simulink model "SynthFSE"  (R2023a)
settings: Solver=ode45  StartTime=0.0  StopTime=1780  RelTol=1e-3  EnableMultiTasking=on
undefined symbols (not defined in the file): j, QAM
libraries: hdlBasic x71, dspmlti4 x2, hdlUtilities x1, vmcUtilities x1
(part 1 of 2)
settings Model: Creator=alexc  LastModifiedBy=robg
settings SolverCC: AlgebraicLoopSolver=TrustRegion
settings DataIOCC: LimitDataPoints=on  SaveFormat=Array  SignalLoggingSaveFormat=ModelDataLogs  ReturnWorkspaceOutputs=off  SignalLoggingName=sigsOut
settings OptimizationCC: BlockReduction=off  BooleanDataType=off  ExpressionDepthLimit=2147483647  InitFltsAndDblsToZero=on  LifeSpan=inf
settings DebuggingCC: SaveWithParameterizedLinksMsg=none  UnderspecifiedInitializationDetection=Classic  MergeDetectMultiDrivingBlocksExec=none  SignalResolutionControl=TryResolveAllWithWarning  MultiTaskDSMMsg=warning  MultiTaskCondExecSysMsg=none  FcnCallInpInsideContextMsg=warning  UnconnectedInputMsg=warning  UnconnectedOutputMsg=warning  UnconnectedLineMsg=warning  StateNameClashWarn=warning  SFUnexpectedBacktrackingDiag=warning  SFNoUnconditionalDefaultTransitionDiag=warning  SFExecutionAtInitializationDiag=none  ArithmeticOperatorsInVariantConditions=warning
settings HardwareCC: ProdBitPerPointer=32  ProdBitPerSizeT=32  ProdBitPerPtrDiffT=32  ProdLargestAtomicFloat=None  ProdIntDivRoundTo=Undefined  ProdEndianess=Unspecified  ProdWordSize=32  ProdHWDeviceType=32-bit Generic  TargetUnknown=on
settings ModelReferenceCC: EnableRefExpFcnMdlSchedulingChecks=on  PropagateSignalLabelsOutOfModel=off
settings SFSimCC: SimUseLocalCustomCode=off  CustomCodeUndefinedFunction=UseInterfaceOnly
settings RTWCC: RTWUseLocalCustomCode=off  DLArmComputeVersion=19.05
settings CodeAppCC: StateflowObjectComments=on
settings GRTTargetCC: TargetFcnLib=ansi_tfl_tmw.mat  TargetLangStandard=C89/C90 (ANSI)  CombineOutputUpdateFcns=off  GRTInterface=on
settings ConfigComp: CovMetricSettings=dw  CovSaveCumulativeToWorkspaceVar=on  CovSaveSingleToWorkspaceVar=on  CovExternalEMLEnable=off

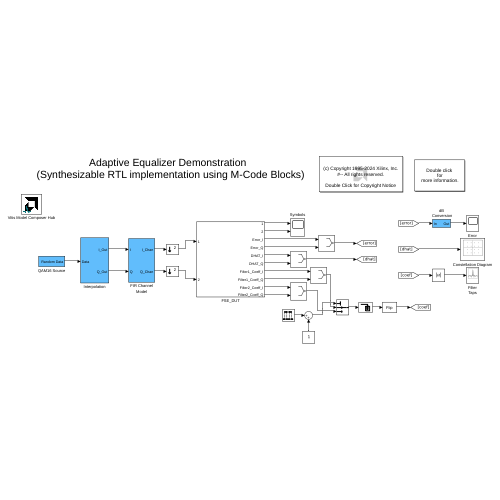
[thumbnail: Simulink's stored preview of the top-level diagram]
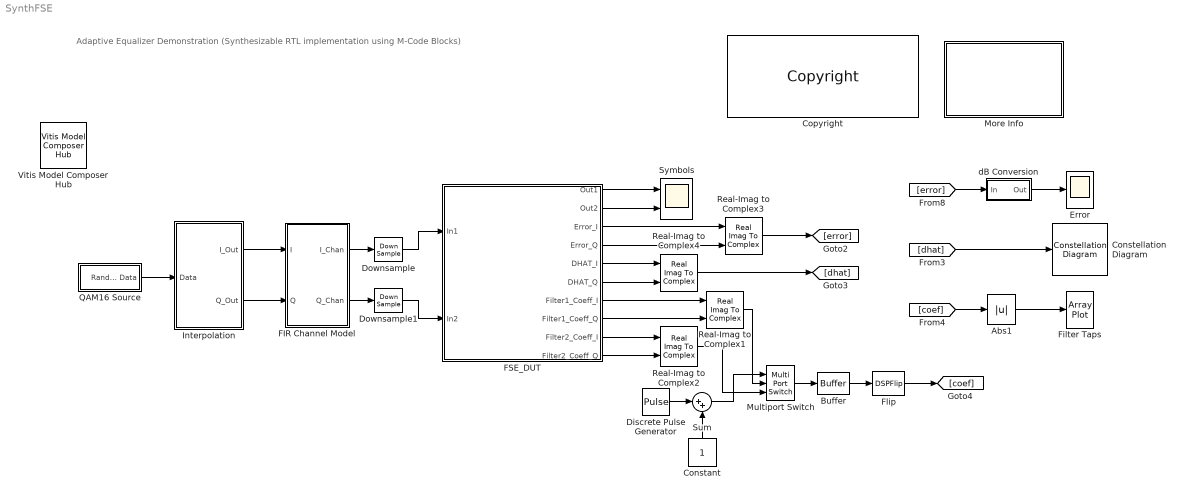
== system SynthFSE ==
  note: Adaptive Equalizer Demonstration
      | (Synthesizable RTL implementation using M-Code Blocks)
  Abs1 : Abs
  Buffer : Buffer  N=8
  Constant : Constant
  Constellation Diagram : ConstellationDiagram  WindowPosition=[288.000000,26.000000,474.000000,337.000000,]  ScopeFrameLocation=window  SymbolsToDisplaySource=Property  SymbolsToDisplay=1000  ReferenceConstellation=16-QAM  YLimits=[-1.8578 1.8744]  ColorFading=on  DefaultConfigurationName=comm.scopes.ConstellationDiagramBlockCfg
  Copyright : hdlUtilities/Copyright  copyrighttext="Copyright (c) 2024  by  Xilinx, Inc. All rights reserved.<br><br>This file contains proprietary, confidential information of Xilinx, Inc., is distributed under license from Xilinx, Inc., and may be used, copied and/or disclosed only pursuant to the terms of a valid license agreement with Xilinx, Inc. Xilinx hereby grants you a license to use this file solely for design, simulation, implementation and creation of design files limited to Xilinx devices or technologies. Use with non-Xilinx devices or technologies is expressly prohibited and immediately terminates your license unless covered by a separate agreement.<br><br>Xilinx is providing this design, code, or information \"as-is\" solely for use in developing programs and solutions for Xilinx devices, with no obligation on the part of Xilinx to provide support. By providing this design, code, or information as one possible implementation of this feature, application or standard, Xilinx is making no representation that this implementation is free from any claims of infringement. You are responsible for obtaining any rights you may require for your implementation. Xilinx expressly disclaims any warranty whatsoever with respect to the adequacy of the implementation, including but not limited to any warranties or representations that this implementation is free from claims of infringement, implied warranties of merchantability or fitness for a particular purpose.<br><br>Xilinx products are not intended for use in life support appliances, devices, or systems. Use in such applications is expressly prohibited.<br><br>Any modifications that are made to the Source Code are done at the user's sole risk and will be unsupported.<br><br>This copyright and support notice must be retained as part of this text at all times. (c) Copyright 1995-2024 Xilinx, Inc. All rights reserved."  block_type=copyright
  Discrete Pulse Generator : DiscretePulseGenerator  SampleTime=.5
  Downsample : DownSample  RateOptions=Allow multirate processing
  Downsample1 : DownSample  RateOptions=Allow multirate processing
  Error : Scope
  FIR Channel Model : Subsystem  mask{chan=[1+j*0.1 .2 j*0.2 0 0 0 0 0 0 0]}
      mask prompts: chan "Channel"
  FSE_DUT : Subsystem
  Filter Taps : ArrayPlot  WindowPosition=[66.000000,260.000000,329.000000,270.000000,]  ScopeFrameLocation=window  PlotType=Line  AxesScaling=Manual  MaximizeAxes=On  XLabel=Samples  YLabel=Filter Coefficients  YLimits=[0.005979,1.0369]  DefaultConfigurationName=dsp.scopes.ArrayPlotBlockSpecification
  Flip : DSPFlip
  Interpolation : Subsystem
  More Info : Subsystem
      mask Display: disp('Double click\n for\n more information.')
  Multiport Switch : MultiPortSwitch  Inputs=2
  QAM16 Source : Subsystem
  Real-Imag to Complex{1..4} (4 alike) : RealImagToComplex
  Sum : Sum  Inputs=|++  InputSameDT=on  SaturateOnIntegerOverflow=on  OutDataTypeStr=Inherit: Same as first input
  Symbols : Scope  NumInputPorts=2
  Vitis Model Composer Hub : vmcUtilities/Vitis Model Composer Hub  Tag=genX  CodeGeneration=off  SubsystemName=FSE_DUT  CompilationType=HDLCompilation  SubsystemType=HDLNode  ExportTypeV2=IP Catalog  StartColumn=1  NumberOfColumns=1  TargetDirectory=./netlist  exportDesign=on  analyzeDesign=off  validateDesignOnHw=off  ExportType=System Generator  IpVendor=xilinx.com  IpLibrary=hls  IpVersion=1.0  IpHWLanguage=Verilog  AieCompilerOptions={}  AieSimulatorOptions={}  CreateTestbench=off  TestbenchStackSize=10  RunRtlSim=off  RunCSim=off  RunAieSim=off  AieSimTimeout=50000  RunAieSimProfiling=off  LaunchVitisAnalyzer=off  PlotOutput=off  RunX86Sim=off  X86SimTimeout=10  GenHwImage=off  GenLibadfXo=on  GenHwValidationCode=off  PlatformType=Not Specified  HwSystemType=Baremetal  HwValidationTarget=hw  ProjDevice=xcku11p-ffva1156-1-e  ProjDevicePart=xcku11p-ffva1156-1-e  SamplePeriod=-1  ClockFrequency=200  DataPathParallelism=1  xilinxfamily=kintexuplus  part=xcku11p  speed=-1-e  package=ffva1156  directory=./netlist/ip/FSE_DUT/src  testbench=off  incr_netlist=off  synthesis_tool=Vivado  clock_wrapper=Clock Enables  dbl_ovrd=According to Block Masks  dcm_input_clock_period=10  sysclk_period=10  simulink_period=1  eval_field=0  IPInfoJsonString="{\"DUTSubsystemName\":\"FSE_DUT\",\"HDLSubsystem\":{\"SubsystemName\":\"FSE_DUT\",\"IPName\":\"Subsystem\",\"IPLibrary\":\"VMC\",\"IPVendor\":\"User Company\",\"IPVersion\":\"1.0\",\"TargetDirectory\":\"./netlist\",\"SubsystemDir\":\"./netlist/ip/FSE_DUT\",\"FreqHz\":\"100000000\"},\"SubsystemTag\":\"HDLNode\"}"  LogFileName=/group/xcoswmktg2/robg/git/vmc_examples/Vitis_Model_Composer/Examples/HDL/Digital_Filtering/LMS_based_adaptive_Equalization_Synth_RTL/netlist/model_composer.log  NThreads=4  IPConfigFile=/tmp/vmctmp-robg/363/ipconfig.json
  dB Conversion : Subsystem
  wires:
  QAM16 Source/1(" Random Data") -> Interpolation/1(Data)
  Interpolation/2(Q_Out) -> FIR Channel Model/2(Q)
  Interpolation/1(I_Out) -> FIR Channel Model/1(I)
  FIR Channel Model/1(I_Chan) -> Downsample/1
  FIR Channel Model/2(Q_Chan) -> Downsample1/1
  Abs1/1 -> Filter Taps/1
  dB Conversion/1(Out) -> Error/1
  [coef] -> Abs1/1
  [dhat] -> Constellation Diagram/1
  [error] -> dB Conversion/1(In)
  Discrete Pulse Generator/1 -> Sum/1
  Multiport Switch/1 -> Buffer/1
  Flip/1 -> [coef]
  Real-Imag to Complex2/1 -> Multiport Switch/3
  Constant/1 -> Sum/2
  Buffer/1 -> Flip/1
  Sum/1 -> Multiport Switch/1
  Real-Imag to Complex1/1 -> Multiport Switch/2
  Real-Imag to Complex4/1 -> [dhat]
  Real-Imag to Complex3/1 -> [error]
  Downsample/1 -> FSE_DUT/1(In1)
  Downsample1/1 -> FSE_DUT/2(In2)
  FSE_DUT/1(Out1) -> Symbols/1
  FSE_DUT/2(Out2) -> Symbols/2
  FSE_DUT/3(Error_I) -> Real-Imag to Complex3/1
  FSE_DUT/4(Error_Q) -> Real-Imag to Complex3/2
  FSE_DUT/5(DHAT_I) -> Real-Imag to Complex4/1
  FSE_DUT/6(DHAT_Q) -> Real-Imag to Complex4/2
  FSE_DUT/7(Filter1_Coeff_I) -> Real-Imag to Complex1/1
  FSE_DUT/8(Filter1_Coeff_Q) -> Real-Imag to Complex1/2
  FSE_DUT/9(Filter2_Coeff_I) -> Real-Imag to Complex2/1
  FSE_DUT/10(Filter2_Coeff_Q) -> Real-Imag to Complex2/2

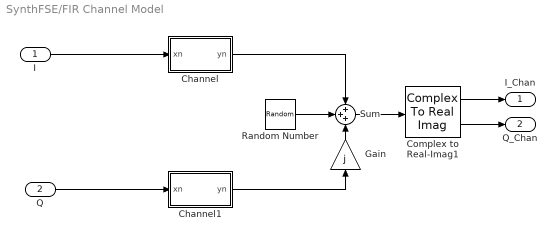
== system SynthFSE/FIR Channel Model ==
  I : Inport
  Q : Inport  Port=2
  Channel : Subsystem
  Channel1 : Subsystem
  Complex to Real-Imag1 : ComplexToRealImag
  Gain : Gain  Gain=j  SaturateOnIntegerOverflow=on  OutDataTypeStr=Inherit: Same as input  ParamDataTypeStr=Inherit: Same as input
  Random Number : RandomNumber  Variance=.01  SampleTime=100000
  Sum : Sum  Inputs=+++  InputSameDT=on  SaturateOnIntegerOverflow=on  OutDataTypeStr=Inherit: Same as first input
  I_Chan : Outport  VectorParamsAs1DForOutWhenUnconnected=off
  Q_Chan : Outport  Port=2  VectorParamsAs1DForOutWhenUnconnected=off
  wires:
  Channel1/1(yn) -> Gain/1
  Channel/1(yn) -> Sum/1
  Q/1 -> Channel1/1(xn)
  I/1 -> Channel/1(xn)
  Random Number/1 -> Sum/2
  Gain/1 -> Sum/3
  Sum/1 -> Complex to Real-Imag1/1
  Complex to Real-Imag1/2 -> Q_Chan/1
  Complex to Real-Imag1/1 -> I_Chan/1

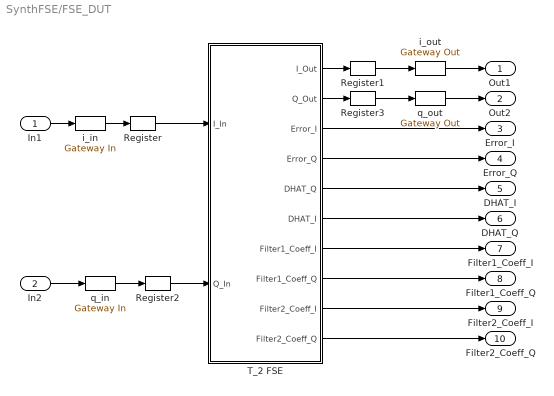
== system SynthFSE/FSE_DUT ==
  In1 : Inport
  In2 : Inport  Port=2
  Register{,1..3} (4 alike) : hdlBasic/Register  init=0  rst=off  en=off  XmcBlockStatus=1  maskContainerNames=tabcontainer1  block_type=register  block_config=sysgen:Register_config
  T_2 FSE : Subsystem  mask{mu=.005}
  i_in : hdlBasic/Gateway In  gui_display_data_type=Fixed-point  arith_type=Signed (2's comp)  n_bits=12  bin_pt=10  preci_type=Single  exp_width=8  frac_width=24  rows=1  columns=1  quantization="Round  (unbiased: +/- Inf)"  overflow=Saturate  period=2  UseAsADC=off  ADCChannel='1'  interface=None  automatic_assignment=on  address_offset=hex2dec('00')  intf_name=''  intf_description=''  default_value=0  timing_constraint=None  locs_specified=off  LOCs={}  io_standard={}  inherit_from_input=off  hdl_port=on  XmcBlockStatus=1  maskContainerNames=group4  block_type=gatewayin  block_config=sysgen:gateway_in_config  block_width_w=590  block_height_w=620  block_width=640  block_height=850
  i_out : hdlBasic/Gateway Out  inherit_from_input=off  hdl_port=on  rows=1  columns=1  UseAsDAC=off  DACChannel='1'  interface=None  automatic_assignment=on  address_offset=hex2dec('00')  intf_name=''  intf_description=''  timing_constraint="Data Rate;  Set 'FAST' Attribute"  locs_specified=off  LOCs={}  io_standard={}  XmcBlockStatus=1  maskContainerNames=group4  block_type=gatewayout  block_config=sysgen:gateway_out_config  block_width_w=590  block_height_w=620  block_width=620  block_height=750
  q_in : hdlBasic/Gateway In  gui_display_data_type=Fixed-point  arith_type=Signed (2's comp)  n_bits=12  bin_pt=10  preci_type=Single  exp_width=8  frac_width=24  rows=1  columns=1  quantization="Round  (unbiased: +/- Inf)"  overflow=Saturate  period=2  UseAsADC=off  ADCChannel='1'  interface=None  automatic_assignment=on  address_offset=hex2dec('00')  intf_name=''  intf_description=''  default_value=0  timing_constraint=None  locs_specified=off  LOCs={}  io_standard={}  inherit_from_input=off  hdl_port=on  XmcBlockStatus=1  maskContainerNames=group4  block_type=gatewayin  block_config=sysgen:gateway_in_config  block_width_w=590  block_height_w=620  block_width=640  block_height=850
  q_out : hdlBasic/Gateway Out  inherit_from_input=off  hdl_port=on  rows=1  columns=1  UseAsDAC=off  DACChannel='1'  interface=None  automatic_assignment=on  address_offset=hex2dec('00')  intf_name=''  intf_description=''  timing_constraint="Data Rate;  Set 'FAST' Attribute"  locs_specified=off  LOCs={}  io_standard={}  XmcBlockStatus=1  maskContainerNames=group4  block_type=gatewayout  block_config=sysgen:gateway_out_config  block_width_w=590  block_height_w=620  block_width=620  block_height=750
  Out1 : Outport
  Out2 : Outport  Port=2
  Error_I : Outport  Port=3
  Error_Q : Outport  Port=4
  DHAT_I : Outport  Port=5
  DHAT_Q : Outport  Port=6
  Filter1_Coeff_I : Outport  Port=7
  Filter1_Coeff_Q : Outport  Port=8
  Filter2_Coeff_I : Outport  Port=9
  Filter2_Coeff_Q : Outport  Port=10
  wires:
  T_2 FSE/5(DHAT_Q) -> DHAT_I/1
  Register/1 -> T_2 FSE/1(I_In)
  T_2 FSE/7(Filter1_Coeff_I) -> Filter1_Coeff_I/1
  T_2 FSE/8(Filter1_Coeff_Q) -> Filter1_Coeff_Q/1
  T_2 FSE/2(Q_Out) -> Register3/1
  Register3/1 -> q_out/1
  i_in/1 -> Register/1
  Register1/1 -> i_out/1
  T_2 FSE/3(Error_I) -> Error_I/1
  T_2 FSE/4(Error_Q) -> Error_Q/1
  q_out/1 -> Out2/1
  T_2 FSE/6(DHAT_I) -> DHAT_Q/1
  T_2 FSE/9(Filter2_Coeff_I) -> Filter2_Coeff_I/1
  q_in/1 -> Register2/1
  i_out/1 -> Out1/1
  T_2 FSE/10(Filter2_Coeff_Q) -> Filter2_Coeff_Q/1
  Register2/1 -> T_2 FSE/2(Q_In)
  In2/1 -> q_in/1
  In1/1 -> i_in/1
  T_2 FSE/1(I_Out) -> Register1/1

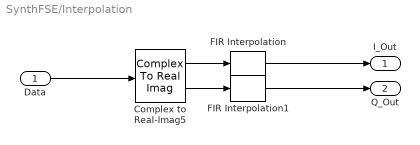
== system SynthFSE/Interpolation ==
  Data : Inport
  Complex to Real-Imag5 : ComplexToRealImag
  FIR Interpolation : dspmlti4/FIR Interpolation  FilterSource=Dialog parameters  PrivateCoeffs=0  h=sinc(-3:.25:3);  L=4  FilterObject=Hm_firinterp  framing=Allow multirate processing  outputBufInitCond=0  roundingMode=Floor  overflowMode=off  firstCoeffDataTypeStr=Inherit: Same word length as input  firstCoeffMin=[]  firstCoeffMax=[]  firstCoeffLastDataTypeStr=Inherit: Same word length as input  outputDataTypeStr=Inherit: Same as accumulator  outputMin=[]  outputMax=[]  outputLastDataTypeStr=Inherit: Same as accumulator
  FIR Interpolation1 : dspmlti4/FIR Interpolation  FilterSource=Dialog parameters  PrivateCoeffs=0  h=sinc(-3:.25:3);  L=4  FilterObject=Hm_firinterp  framing=Allow multirate processing  outputBufInitCond=0  roundingMode=Floor  overflowMode=off  firstCoeffDataTypeStr=Inherit: Same word length as input  firstCoeffMin=[]  firstCoeffMax=[]  firstCoeffLastDataTypeStr=Inherit: Same word length as input  outputDataTypeStr=Inherit: Same as accumulator  outputMin=[]  outputMax=[]  outputLastDataTypeStr=Inherit: Same as accumulator
  I_Out : Outport  VectorParamsAs1DForOutWhenUnconnected=off
  Q_Out : Outport  Port=2  VectorParamsAs1DForOutWhenUnconnected=off
  wires:
  Complex to Real-Imag5/2 -> FIR Interpolation1/1
  Complex to Real-Imag5/1 -> FIR Interpolation/1
  FIR Interpolation/1 -> I_Out/1
  Data/1 -> Complex to Real-Imag5/1
  FIR Interpolation1/1 -> Q_Out/1

== system SynthFSE/More Info ==
  note: This design shows a T/2 adaptive Fractionally Space Equalizer (FSE)
      | operating on a 16-QAM data source with noise and filtering introduced
      | in the channel model.  The two 4-tap FIR filters are based on an
      | SRL16E-based MAC implementation.
      |
      | The DHAT scope provides an X-Y plot of the I and Q filter outputs from
      | within the FSE.  As the simulation progresses, these symbols will
      | converge as the error is reduced.  The magnitude of the filter coefficients
      | is shown in a vector scope as well.  Increasing the simulation duration
      | will allow better visualization of the adaptive FSE effects on the filter output.
      |
      | For additional information on FSE:
      |
      | J.R. Treichler, I. Fijalkow, and C.R. Johnson, Jr.  "Fractionally Spaced
      | Equalizers"  IEEE Signal Processing Magazine, May 1996, pp. 65-81.
      |
      | Chris H. Dick, "Design and implementation of high-performance FPGA
      | signal processing datapaths for software-defined radios" VMEbus
      | Systems, August 2001.
  note: Adaptive FSE Demonstration Using a 16-QAM Source

== system SynthFSE/QAM16 Source ==
  QAM16 - I : Subsystem
  QAM16 -Q : Subsystem
  Real-Imag to Complex : RealImagToComplex
  " Random Data" : Outport  VectorParamsAs1DForOutWhenUnconnected=off
  wires:
  QAM16 - I/1(I) -> Real-Imag to Complex/1
  QAM16 -Q/1(Q) -> Real-Imag to Complex/2
  Real-Imag to Complex/1 -> " Random Data"/1

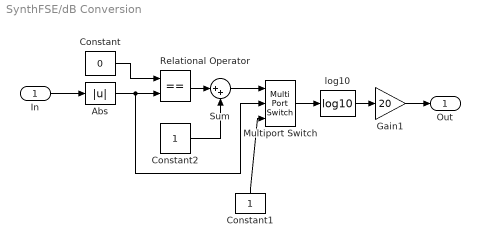
== system SynthFSE/dB Conversion ==
  In : Inport
  Abs : Abs
  Constant : Constant  Value=0
  Constant1 : Constant
  Constant2 : Constant
  Gain1 : Gain  Gain=20  SaturateOnIntegerOverflow=on  OutDataTypeStr=Inherit: Same as input  ParamDataTypeStr=Inherit: Same as input
  Multiport Switch : MultiPortSwitch  Inputs=2
  Relational Operator : RelationalOperator  Operator===
  Sum : Sum  Inputs=|++  InputSameDT=on  SaturateOnIntegerOverflow=on  OutDataTypeStr=Inherit: Same as first input
  log10 : Math  Operator=log10  SignedPower=on
  Out : Outport  VectorParamsAs1DForOutWhenUnconnected=off
  wires:
  Multiport Switch/1 -> log10/1
  Constant1/1 -> Multiport Switch/3
  Constant/1 -> Relational Operator/1
  Abs/1 -> Multiport Switch/2, Relational Operator/2
  Constant2/1 -> Sum/2
  Sum/1 -> Multiport Switch/1
  Relational Operator/1 -> Sum/1
  Gain1/1 -> Out/1
  In/1 -> Abs/1
  log10/1 -> Gain1/1

== system SynthFSE/FIR Channel Model/Channel ==
  xn : Inport
  Chan Re : Subsystem
  yn : Outport  VectorParamsAs1DForOutWhenUnconnected=off
  wires:
  xn/1 -> Chan Re/1(Input)
  Chan Re/1(Output) -> yn/1

== system SynthFSE/FIR Channel Model/Channel1 ==
  xn : Inport
  Chan Re : Subsystem
  yn : Outport  VectorParamsAs1DForOutWhenUnconnected=off
  wires:
  xn/1 -> Chan Re/1(Input)
  Chan Re/1(Output) -> yn/1

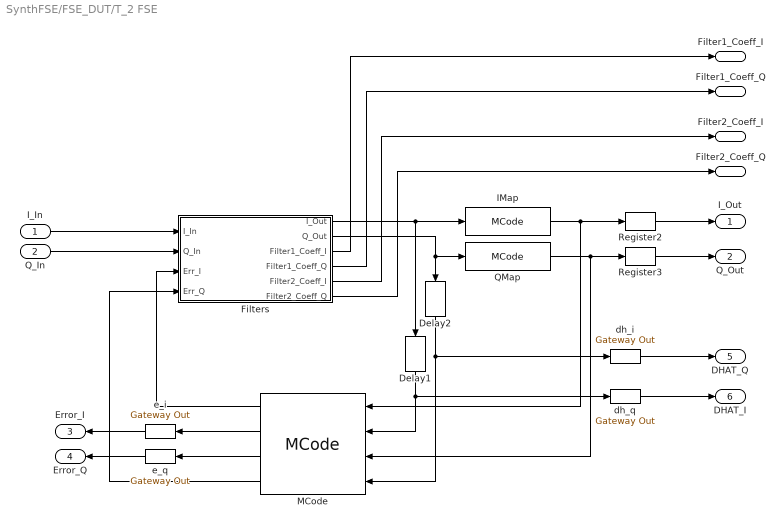
== system SynthFSE/FSE_DUT/T_2 FSE ==
  I_In : Inport
  Q_In : Inport  Port=2
  Delay1 : hdlBasic/Delay  rst=off  en=off  latency=2  reg_retiming=on  XmcBlockStatus=1  maskContainerNames=group1  block_type=delay  block_config=sysgen:Delay_config
  Delay2 : hdlBasic/Delay  rst=off  en=off  latency=2  reg_retiming=on  XmcBlockStatus=1  maskContainerNames=group1  block_type=delay  block_config=sysgen:Delay_config
  Filters : Subsystem
  IMap : hdlBasic/MCode  mfname=QAM4map  explicit_period=off  period=1  iptable={'i',''}  optable={'v','off'}  enable_stdout=off  enable_debug=off  suppress_output=off  defparams={}  hide_port_list={}  block_type=mcode  block_width=444  block_height=788
      settings: infoedit=Pass input values to a MATLAB function for evaluation in Xilinx fixed-point type. The input ports of the block are input arguments of the function. The output ports of the block are output arguments of the function.  block_version=8.1
  MCode : hdlBasic/MCode  mfname=lmsErr  explicit_period=off  period=1  iptable={'sym_i','';'filt_i','';'sym_q','';'filt_q','';'mu','mu'}  optable={'mu_e_i','off';'e_i','off';'e_q','off';'mu_e_q','off'}  enable_stdout=off  enable_debug=off  suppress_output=1  defparams={'mu',mu}  hide_port_list={}  block_type=mcode  block_width=444  block_height=788
      settings: infoedit=Pass input values to a MATLAB function for evaluation in Xilinx fixed-point type. The input ports of the block are input arguments of the function. The output ports of the block are output arguments of the function.  block_version=8.2.EA1
  QMap : hdlBasic/MCode  mfname=QAM4map  explicit_period=off  period=1  iptable={'i',''}  optable={'v','off'}  enable_stdout=off  enable_debug=off  suppress_output=off  defparams={}  hide_port_list={}  block_type=mcode  block_width=444  block_height=788
      settings: infoedit=Pass input values to a MATLAB function for evaluation in Xilinx fixed-point type. The input ports of the block are input arguments of the function. The output ports of the block are output arguments of the function.  block_version=8.1
  Register2 : hdlBasic/Register  init=0  rst=off  en=off  XmcBlockStatus=1  maskContainerNames=tabcontainer1  block_type=register  block_config=sysgen:Register_config
  Register3 : hdlBasic/Register  init=0  rst=off  en=off  XmcBlockStatus=1  maskContainerNames=tabcontainer1  block_type=register  block_config=sysgen:Register_config
  dh_i : hdlBasic/Gateway Out  inherit_from_input=off  hdl_port=off  rows=1  columns=1  UseAsDAC=off  DACChannel='1'  interface=None  automatic_assignment=on  address_offset=hex2dec('00')  intf_name=''  intf_description=''  timing_constraint=None  locs_specified=off  LOCs={}  io_standard={}  XmcBlockStatus=1  maskContainerNames=group4  block_type=gatewayout  block_config=sysgen:gateway_out_config  block_width_w=590  block_height_w=620  block_width=620  block_height=750
  dh_q : hdlBasic/Gateway Out  inherit_from_input=off  hdl_port=off  rows=1  columns=1  UseAsDAC=off  DACChannel='1'  interface=None  automatic_assignment=on  address_offset=hex2dec('00')  intf_name=''  intf_description=''  timing_constraint=None  locs_specified=off  LOCs={}  io_standard={}  XmcBlockStatus=1  maskContainerNames=group4  block_type=gatewayout  block_config=sysgen:gateway_out_config  block_width_w=590  block_height_w=620  block_width=620  block_height=750
  e_i : hdlBasic/Gateway Out  inherit_from_input=off  hdl_port=off  rows=1  columns=1  UseAsDAC=off  DACChannel='1'  interface=None  automatic_assignment=on  address_offset=hex2dec('00')  intf_name=''  intf_description=''  timing_constraint=None  locs_specified=off  LOCs={}  io_standard={}  XmcBlockStatus=1  maskContainerNames=group4  block_type=gatewayout  block_config=sysgen:gateway_out_config  block_width_w=590  block_height_w=620  block_width=620  block_height=750
  e_q : hdlBasic/Gateway Out  inherit_from_input=off  hdl_port=off  rows=1  columns=1  UseAsDAC=off  DACChannel='1'  interface=None  automatic_assignment=on  address_offset=hex2dec('00')  intf_name=''  intf_description=''  timing_constraint=None  locs_specified=off  LOCs={}  io_standard={}  XmcBlockStatus=1  maskContainerNames=group4  block_type=gatewayout  block_config=sysgen:gateway_out_config  block_width_w=590  block_height_w=620  block_width=620  block_height=750
  I_Out : Outport  VectorParamsAs1DForOutWhenUnconnected=off
  Q_Out : Outport  Port=2  VectorParamsAs1DForOutWhenUnconnected=off
  Error_I : Outport  Port=3  VectorParamsAs1DForOutWhenUnconnected=off
  Error_Q : Outport  Port=4  VectorParamsAs1DForOutWhenUnconnected=off
  DHAT_Q : Outport  Port=5  VectorParamsAs1DForOutWhenUnconnected=off
  DHAT_I : Outport  Port=6  VectorParamsAs1DForOutWhenUnconnected=off
  Filter1_Coeff_I : Outport  Port=7  VectorParamsAs1DForOutWhenUnconnected=off
  Filter1_Coeff_Q : Outport  Port=8  VectorParamsAs1DForOutWhenUnconnected=off
  Filter2_Coeff_I : Outport  Port=9  VectorParamsAs1DForOutWhenUnconnected=off
  Filter2_Coeff_Q : Outport  Port=10  VectorParamsAs1DForOutWhenUnconnected=off
  wires:
  Q_In/1 -> Filters/2(Q_In)
  Filters/1(I_Out) -> Delay1/1, IMap/1
  QMap/1 -> Register3/1, MCode/3
  IMap/1 -> Register2/1, MCode/1
  Filters/2(Q_Out) -> Delay2/1, QMap/1
  I_In/1 -> Filters/1(I_In)
  Delay1/1 -> dh_q/1, MCode/2
  Delay2/1 -> MCode/4, dh_i/1
  dh_i/1 -> DHAT_Q/1
  dh_q/1 -> DHAT_I/1
  Register2/1 -> I_Out/1
  Register3/1 -> Q_Out/1
  e_q/1 -> Error_Q/1
  MCode/2 -> e_i/1
  MCode/3 -> e_q/1
  e_i/1 -> Error_I/1
  MCode/1 -> Filters/3(Err_I)
  MCode/4 -> Filters/4(Err_Q)
  Filters/3(Filter1_Coeff_I) -> Filter1_Coeff_I/1
  Filters/4(Filter1_Coeff_Q) -> Filter1_Coeff_Q/1
  Filters/5(Filter2_Coeff_I) -> Filter2_Coeff_I/1
  Filters/6(Filter2_Coeff_Q) -> Filter2_Coeff_Q/1

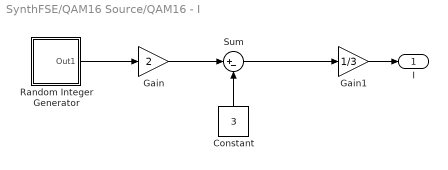
== system SynthFSE/QAM16 Source/QAM16 - I ==
  Constant : Constant  Value=3
  Gain : Gain  Gain=2  SaturateOnIntegerOverflow=on  OutDataTypeStr=Inherit: Same as input  ParamDataTypeStr=Inherit: Same as input
  Gain1 : Gain  Gain=1/3  SaturateOnIntegerOverflow=on  OutDataTypeStr=Inherit: Same as input  ParamDataTypeStr=Inherit: Same as input
  Random Integer Generator : Subsystem  mask{M=4, seed=1, Ts=4}
      mask prompts: M "M-ary Number"; seed "Initial seed"; Ts "Sample Time"
  Sum : Sum  Inputs=|+-  InputSameDT=on  SaturateOnIntegerOverflow=on  OutDataTypeStr=Inherit: Same as first input
  I : Outport  VectorParamsAs1DForOutWhenUnconnected=off
  wires:
  Random Integer Generator/1(Out1) -> Gain/1
  Gain/1 -> Sum/1
  Constant/1 -> Sum/2
  Sum/1 -> Gain1/1
  Gain1/1 -> I/1

== system SynthFSE/QAM16 Source/QAM16 -Q ==
  Constant : Constant  Value=3
  Gain : Gain  Gain=2  SaturateOnIntegerOverflow=on  OutDataTypeStr=Inherit: Same as input  ParamDataTypeStr=Inherit: Same as input
  Gain1 : Gain  Gain=1/3  SaturateOnIntegerOverflow=on  OutDataTypeStr=Inherit: Same as input  ParamDataTypeStr=Inherit: Same as input
  Random Integer Generator : Subsystem  mask{M=4, seed=4, Ts=4}
      mask prompts: M "M-ary Number"; seed "Initial seed"; Ts "Sample Time"
  Sum : Sum  Inputs=|+-  InputSameDT=on  SaturateOnIntegerOverflow=on  OutDataTypeStr=Inherit: Same as first input
  Q : Outport  VectorParamsAs1DForOutWhenUnconnected=off
  wires:
  Random Integer Generator/1(Out1) -> Gain/1
  Gain/1 -> Sum/1
  Constant/1 -> Sum/2
  Sum/1 -> Gain1/1
  Gain1/1 -> Q/1

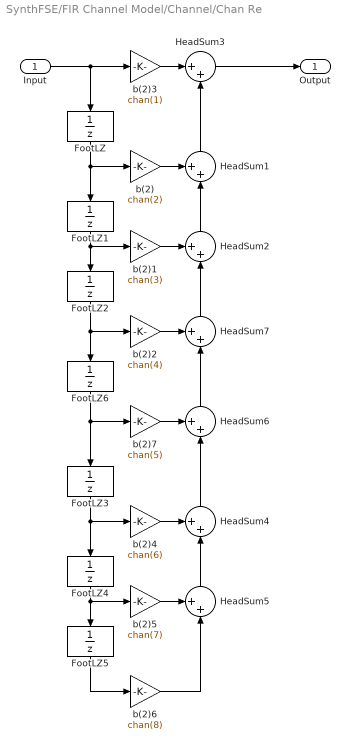
== system SynthFSE/FIR Channel Model/Channel/Chan Re ==
  Input : Inport
  FootLZ : UnitDelay  HasFrameUpgradeWarning=on
  FootLZ{1..2,4..6} (5 alike) : UnitDelay  SampleTime=-1  HasFrameUpgradeWarning=on
  FootLZ3 : UnitDelay  HasFrameUpgradeWarning=on
  HeadSum{1..2,4..7} (6 alike) : Sum  Inputs=++|  InputSameDT=on  SaturateOnIntegerOverflow=on  OutDataTypeStr=Inherit: Same as first input
  HeadSum3 : Sum  Inputs=|++  InputSameDT=on  SaturateOnIntegerOverflow=on  OutDataTypeStr=Inherit: Same as first input
  b(2) : Gain  Gain=chan(2)  SaturateOnIntegerOverflow=on  OutDataTypeStr=Inherit: Same as input  ParamDataTypeStr=Inherit: Same as input
  b(2)1 : Gain  Gain=chan(3)  SaturateOnIntegerOverflow=on  OutDataTypeStr=Inherit: Same as input  ParamDataTypeStr=Inherit: Same as input
  b(2)2 : Gain  Gain=chan(4)  SaturateOnIntegerOverflow=on  OutDataTypeStr=Inherit: Same as input  ParamDataTypeStr=Inherit: Same as input
  b(2)3 : Gain  Gain=chan(1)  SaturateOnIntegerOverflow=on  OutDataTypeStr=Inherit: Same as input  ParamDataTypeStr=Inherit: Same as input
  b(2)4 : Gain  Gain=chan(6)  SaturateOnIntegerOverflow=on  OutDataTypeStr=Inherit: Same as input  ParamDataTypeStr=Inherit: Same as input
  b(2)5 : Gain  Gain=chan(7)  SaturateOnIntegerOverflow=on  OutDataTypeStr=Inherit: Same as input  ParamDataTypeStr=Inherit: Same as input
  b(2)6 : Gain  Gain=chan(8)  SaturateOnIntegerOverflow=on  OutDataTypeStr=Inherit: Same as input  ParamDataTypeStr=Inherit: Same as input
  b(2)7 : Gain  Gain=chan(5)  SaturateOnIntegerOverflow=on  OutDataTypeStr=Inherit: Same as input  ParamDataTypeStr=Inherit: Same as input
  Output : Outport  VectorParamsAs1DForOutWhenUnconnected=off
  wires:
  HeadSum6/1 -> HeadSum7/2
  HeadSum4/1 -> HeadSum6/2
  HeadSum7/1 -> HeadSum2/2
  b(2)2/1 -> HeadSum7/1
  FootLZ6/1 -> FootLZ3/1, b(2)7/1
  FootLZ3/1 -> b(2)4/1, FootLZ4/1
  FootLZ4/1 -> FootLZ5/1, b(2)5/1
  FootLZ5/1 -> b(2)6/1
  b(2)4/1 -> HeadSum4/1
  b(2)5/1 -> HeadSum5/1
  HeadSum5/1 -> HeadSum4/2
  b(2)6/1 -> HeadSum5/2
  b(2)7/1 -> HeadSum6/1
  FootLZ2/1 -> FootLZ6/1, b(2)2/1
  FootLZ/1 -> b(2)/1, FootLZ1/1
  FootLZ1/1 -> FootLZ2/1, b(2)1/1
  b(2)/1 -> HeadSum1/1
  b(2)1/1 -> HeadSum2/1
  HeadSum2/1 -> HeadSum1/2
  Input/1 -> FootLZ/1, b(2)3/1
  b(2)3/1 -> HeadSum3/1
  HeadSum1/1 -> HeadSum3/2
  HeadSum3/1 -> Output/1

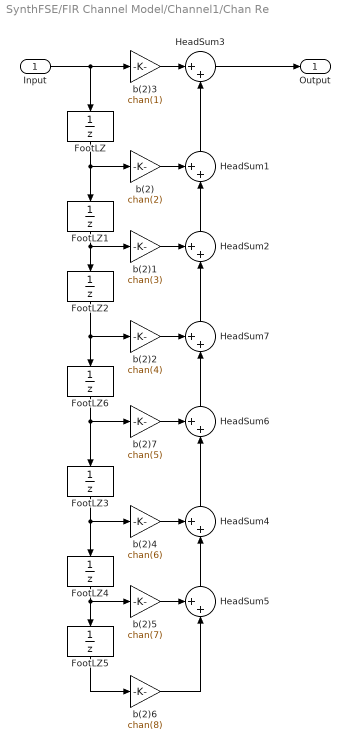
== system SynthFSE/FIR Channel Model/Channel1/Chan Re ==
  Input : Inport
  FootLZ : UnitDelay  HasFrameUpgradeWarning=on
  FootLZ{1..2,4..6} (5 alike) : UnitDelay  SampleTime=-1  HasFrameUpgradeWarning=on
  FootLZ3 : UnitDelay  HasFrameUpgradeWarning=on
  HeadSum{1..2,4..7} (6 alike) : Sum  Inputs=++|  InputSameDT=on  SaturateOnIntegerOverflow=on  OutDataTypeStr=Inherit: Same as first input
  HeadSum3 : Sum  Inputs=|++  InputSameDT=on  SaturateOnIntegerOverflow=on  OutDataTypeStr=Inherit: Same as first input
  b(2) : Gain  Gain=chan(2)  SaturateOnIntegerOverflow=on  OutDataTypeStr=Inherit: Same as input  ParamDataTypeStr=Inherit: Same as input
  b(2)1 : Gain  Gain=chan(3)  SaturateOnIntegerOverflow=on  OutDataTypeStr=Inherit: Same as input  ParamDataTypeStr=Inherit: Same as input
  b(2)2 : Gain  Gain=chan(4)  SaturateOnIntegerOverflow=on  OutDataTypeStr=Inherit: Same as input  ParamDataTypeStr=Inherit: Same as input
  b(2)3 : Gain  Gain=chan(1)  SaturateOnIntegerOverflow=on  OutDataTypeStr=Inherit: Same as input  ParamDataTypeStr=Inherit: Same as input
  b(2)4 : Gain  Gain=chan(6)  SaturateOnIntegerOverflow=on  OutDataTypeStr=Inherit: Same as input  ParamDataTypeStr=Inherit: Same as input
  b(2)5 : Gain  Gain=chan(7)  SaturateOnIntegerOverflow=on  OutDataTypeStr=Inherit: Same as input  ParamDataTypeStr=Inherit: Same as input
  b(2)6 : Gain  Gain=chan(8)  SaturateOnIntegerOverflow=on  OutDataTypeStr=Inherit: Same as input  ParamDataTypeStr=Inherit: Same as input
  b(2)7 : Gain  Gain=chan(5)  SaturateOnIntegerOverflow=on  OutDataTypeStr=Inherit: Same as input  ParamDataTypeStr=Inherit: Same as input
  Output : Outport  VectorParamsAs1DForOutWhenUnconnected=off
  wires:
  b(2)2/1 -> HeadSum7/1
  HeadSum7/1 -> HeadSum2/2
  HeadSum6/1 -> HeadSum7/2
  FootLZ6/1 -> b(2)7/1, FootLZ3/1
  FootLZ2/1 -> FootLZ6/1, b(2)2/1
  FootLZ3/1 -> b(2)4/1, FootLZ4/1
  FootLZ4/1 -> FootLZ5/1, b(2)5/1
  FootLZ5/1 -> b(2)6/1
  b(2)4/1 -> HeadSum4/1
  b(2)5/1 -> HeadSum5/1
  HeadSum5/1 -> HeadSum4/2
  b(2)6/1 -> HeadSum5/2
  b(2)7/1 -> HeadSum6/1
  HeadSum4/1 -> HeadSum6/2
  FootLZ/1 -> b(2)/1, FootLZ1/1
  FootLZ1/1 -> FootLZ2/1, b(2)1/1
  b(2)/1 -> HeadSum1/1
  b(2)1/1 -> HeadSum2/1
  HeadSum2/1 -> HeadSum1/2
  Input/1 -> FootLZ/1, b(2)3/1
  b(2)3/1 -> HeadSum3/1
  HeadSum1/1 -> HeadSum3/2
  HeadSum3/1 -> Output/1

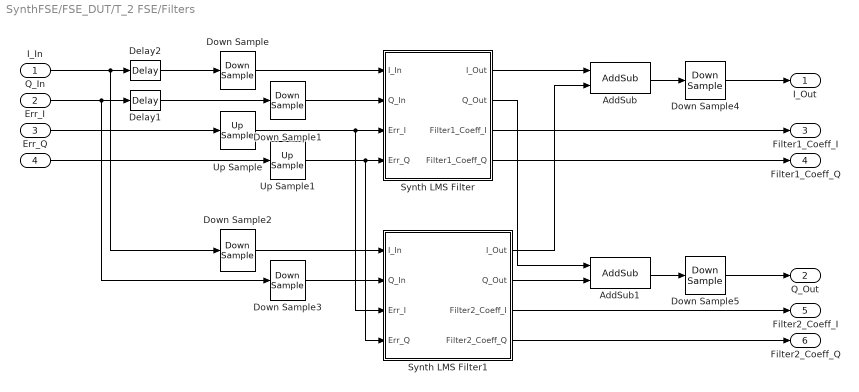
== system SynthFSE/FSE_DUT/T_2 FSE/Filters ==
  I_In : Inport
  Q_In : Inport  Port=2
  Err_I : Inport  Port=3
  Err_Q : Inport  Port=4
  AddSub : hdlBasic/AddSub  mode=Addition  use_carryin=off  use_carryout=off  en=off  latency=0  precision=User Defined  arith_type="Signed  (2's comp)"  n_bits=18  bin_pt=10  quantization=Truncate  overflow=Wrap  use_behavioral_HDL=on  hw_selection=Fabric  pipelined=off  use_rpm=on  XmcBlockStatus=1  maskContainerNames=tabcontainer1  block_type=addsub  block_config=sysgen:Addsub_config
  AddSub1 : hdlBasic/AddSub  mode=Addition  use_carryin=off  use_carryout=off  en=off  latency=0  precision=User Defined  arith_type="Signed  (2's comp)"  n_bits=18  bin_pt=10  quantization=Truncate  overflow=Wrap  use_behavioral_HDL=on  hw_selection=Fabric  pipelined=off  use_rpm=on  XmcBlockStatus=1  maskContainerNames=tabcontainer1  block_type=addsub  block_config=sysgen:Addsub_config
  Delay1 : hdlBasic/Delay  rst=off  en=off  latency=1  reg_retiming=on  XmcBlockStatus=1  maskContainerNames=group1  block_type=delay  block_config=sysgen:Delay_config
  Delay2 : hdlBasic/Delay  rst=off  en=off  latency=1  reg_retiming=on  XmcBlockStatus=1  maskContainerNames=group1  block_type=delay  block_config=sysgen:Delay_config
  Down Sample : hdlBasic/Down Sample  sample_ratio=2  sample_phase="Last Value of Frame  (most efficient)"  en=off  rst=off  latency=1  XmcBlockStatus=1  maskContainerNames=group1  block_type=dsamp  block_config=sysgen:Downsample_config
  Down Sample1 : hdlBasic/Down Sample  sample_ratio=2  sample_phase="Last Value of Frame  (most efficient)"  en=off  rst=off  latency=1  XmcBlockStatus=1  maskContainerNames=group1  block_type=dsamp  block_config=sysgen:Downsample_config
  Down Sample2 : hdlBasic/Down Sample  sample_ratio=2  sample_phase="Last Value of Frame  (most efficient)"  en=off  rst=off  latency=2  XmcBlockStatus=1  maskContainerNames=group1  block_type=dsamp  block_config=sysgen:Downsample_config
  Down Sample3 : hdlBasic/Down Sample  sample_ratio=2  sample_phase="Last Value of Frame  (most efficient)"  en=off  rst=off  latency=2  XmcBlockStatus=1  maskContainerNames=group1  block_type=dsamp  block_config=sysgen:Downsample_config
  Down Sample4 : hdlBasic/Down Sample  sample_ratio=4  sample_phase="Last Value of Frame  (most efficient)"  en=off  rst=off  latency=1  XmcBlockStatus=1  maskContainerNames=group1  block_type=dsamp  block_config=sysgen:Downsample_config
  Down Sample5 : hdlBasic/Down Sample  sample_ratio=4  sample_phase="Last Value of Frame  (most efficient)"  en=off  rst=off  latency=1  XmcBlockStatus=1  maskContainerNames=group1  block_type=dsamp  block_config=sysgen:Downsample_config
  Synth LMS Filter : Subsystem  mask{init_i=[0 0 0 0], init_q=[0 0 0 0]}
      mask prompts: init_i "Init I"; init_q "Init Q"
  Synth LMS Filter1 : Subsystem  mask{init_i=[0 1 0 0], init_q=[0 0 0 0]}
      mask prompts: init_i "Init I"; init_q "Init Q"
  Up Sample : hdlBasic/Up Sample  sample_ratio=4  copy_samples=on  en=off  latency=0  XmcBlockStatus=1  maskContainerNames=group1  block_type=usamp  block_config=sysgen:Upsample_config
  Up Sample1 : hdlBasic/Up Sample  sample_ratio=4  copy_samples=on  en=off  latency=0  XmcBlockStatus=1  maskContainerNames=group1  block_type=usamp  block_config=sysgen:Upsample_config
  I_Out : Outport  VectorParamsAs1DForOutWhenUnconnected=off
  Q_Out : Outport  Port=2  VectorParamsAs1DForOutWhenUnconnected=off
  Filter1_Coeff_I : Outport  Port=3  VectorParamsAs1DForOutWhenUnconnected=off
  Filter1_Coeff_Q : Outport  Port=4  VectorParamsAs1DForOutWhenUnconnected=off
  Filter2_Coeff_I : Outport  Port=5  VectorParamsAs1DForOutWhenUnconnected=off
  Filter2_Coeff_Q : Outport  Port=6  VectorParamsAs1DForOutWhenUnconnected=off
  wires:
  Down Sample3/1 -> Synth LMS Filter1/2(Q_In)
  Down Sample1/1 -> Synth LMS Filter/2(Q_In)
  Down Sample/1 -> Synth LMS Filter/1(I_In)
  AddSub/1 -> Down Sample4/1
  Synth LMS Filter/2(Q_Out) -> AddSub1/1
  Synth LMS Filter1/1(I_Out) -> AddSub/2
  Synth LMS Filter1/2(Q_Out) -> AddSub1/2
  AddSub1/1 -> Down Sample5/1
  Down Sample4/1 -> I_Out/1
  Down Sample5/1 -> Q_Out/1
  Delay2/1 -> Down Sample/1
  Delay1/1 -> Down Sample1/1
  Down Sample2/1 -> Synth LMS Filter1/1(I_In)
  Err_Q/1 -> Up Sample1/1
  Err_I/1 -> Up Sample/1
  Q_In/1 -> Delay1/1, Down Sample3/1
  I_In/1 -> Delay2/1, Down Sample2/1
  Synth LMS Filter/1(I_Out) -> AddSub/1
  Up Sample/1 -> Synth LMS Filter/3(Err_I), Synth LMS Filter1/3(Err_I)
  Up Sample1/1 -> Synth LMS Filter/4(Err_Q), Synth LMS Filter1/4(Err_Q)
  Synth LMS Filter/3(Filter1_Coeff_I) -> Filter1_Coeff_I/1
  Synth LMS Filter/4(Filter1_Coeff_Q) -> Filter1_Coeff_Q/1
  Synth LMS Filter1/3(Filter2_Coeff_I) -> Filter2_Coeff_I/1
  Synth LMS Filter1/4(Filter2_Coeff_Q) -> Filter2_Coeff_Q/1

== system SynthFSE/QAM16 Source/QAM16 - I/Random Integer Generator ==
  Rounding Function : Rounding  Operator=round
  Uniform Random Number : UniformRandomNumber  Minimum=-0.49  Maximum=M-1 + 0.49  Seed=seed  SampleTime=Ts
  Out1 : Outport  VectorParamsAs1DForOutWhenUnconnected=off
  wires:
  Rounding Function/1 -> Out1/1
  Uniform Random Number/1 -> Rounding Function/1

== system SynthFSE/QAM16 Source/QAM16 -Q/Random Integer Generator ==
  Rounding Function : Rounding  Operator=round
  Uniform Random Number : UniformRandomNumber  Minimum=-0.49  Maximum=M-1 + 0.49  Seed=seed  SampleTime=Ts
  Out1 : Outport  VectorParamsAs1DForOutWhenUnconnected=off
  wires:
  Rounding Function/1 -> Out1/1
  Uniform Random Number/1 -> Rounding Function/1

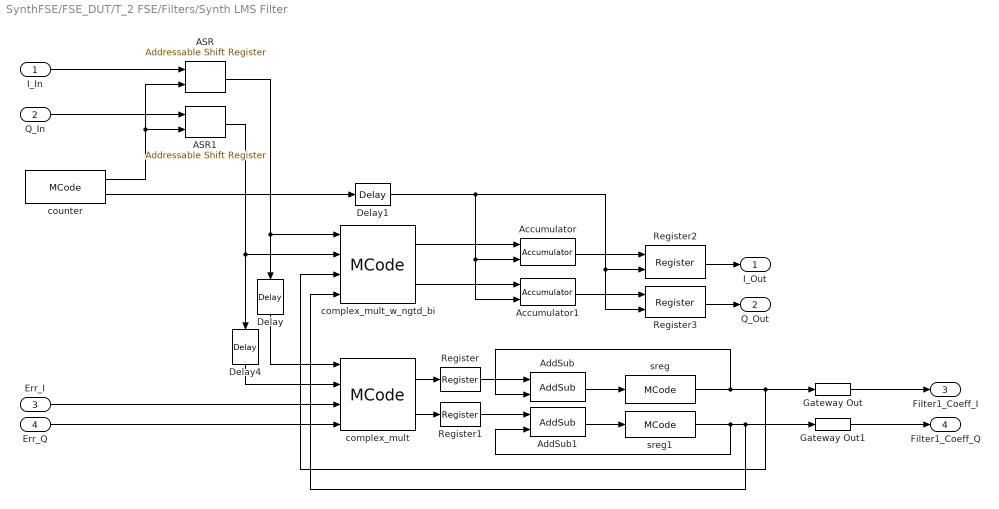
== system SynthFSE/FSE_DUT/T_2 FSE/Filters/Synth LMS Filter ==
  I_In : Inport
  Q_In : Inport  Port=2
  Err_I : Inport  Port=3
  Err_Q : Inport  Port=4
  ASR : hdlBasic/Addressable Shift Register  infer_latency=off  depth=4  initVector=[0]  en=off  use_behavioral_HDL=on  Optimization=Resource  use_rpm=on  XmcBlockStatus=1  maskContainerNames=group1  block_type=addrsr  block_config=sysgen:Addrsr_config
  ASR1 : hdlBasic/Addressable Shift Register  infer_latency=off  depth=4  initVector=[0]  en=off  use_behavioral_HDL=on  Optimization=Resource  use_rpm=on  XmcBlockStatus=1  maskContainerNames=group1  block_type=addrsr  block_config=sysgen:Addrsr_config
  Accumulator : hdlBasic/Accumulator  operation=Add  n_bits=36  overflow=Wrap  scale=1  rst=on  hasbypass=off  en=off  latency=1  msb_inp=100  msb=100  lsb=-100  use_behavioral_HDL=on  implementation=Fabric  XmcBlockStatus=1  maskContainerNames=group3  block_type=accum  block_config=sysgen:Accum_config  block_width=566  block_height=845
  Accumulator1 : hdlBasic/Accumulator  operation=Add  n_bits=36  overflow=Wrap  scale=1  rst=on  hasbypass=off  en=off  latency=1  msb_inp=100  msb=100  lsb=-100  use_behavioral_HDL=on  implementation=Fabric  XmcBlockStatus=1  maskContainerNames=group3  block_type=accum  block_config=sysgen:Accum_config  block_width=566  block_height=845
  AddSub : hdlBasic/AddSub  mode=Addition  use_carryin=off  use_carryout=off  en=off  latency=0  precision=User Defined  arith_type="Signed  (2's comp)"  n_bits=18  bin_pt=10  quantization="Round  (unbiased: +/- Inf)"  overflow=Saturate  use_behavioral_HDL=on  hw_selection=Fabric  pipelined=off  use_rpm=on  XmcBlockStatus=1  maskContainerNames=tabcontainer1  block_type=addsub  block_config=sysgen:Addsub_config
  AddSub1 : hdlBasic/AddSub  mode=Addition  use_carryin=off  use_carryout=off  en=off  latency=0  precision=User Defined  arith_type="Signed  (2's comp)"  n_bits=18  bin_pt=10  quantization="Round  (unbiased: +/- Inf)"  overflow=Saturate  use_behavioral_HDL=on  hw_selection=Fabric  pipelined=off  use_rpm=on  XmcBlockStatus=1  maskContainerNames=tabcontainer1  block_type=addsub  block_config=sysgen:Addsub_config
  Delay : hdlBasic/Delay  rst=off  en=off  latency=27  reg_retiming=off  XmcBlockStatus=1  maskContainerNames=group1  block_type=delay  block_config=sysgen:Delay_config
  Delay1 : hdlBasic/Delay  rst=off  en=off  latency=3  reg_retiming=on  XmcBlockStatus=1  maskContainerNames=group1  block_type=delay  block_config=sysgen:Delay_config
  Delay4 : hdlBasic/Delay  rst=off  en=off  latency=27  reg_retiming=off  XmcBlockStatus=1  maskContainerNames=group1  block_type=delay  block_config=sysgen:Delay_config
  Gateway Out : hdlBasic/Gateway Out  inherit_from_input=off  hdl_port=off  rows=1  columns=1  UseAsDAC=off  DACChannel='1'  interface=None  automatic_assignment=on  address_offset=hex2dec('00')  intf_name=''  intf_description=''  timing_constraint=None  locs_specified=off  LOCs={}  io_standard={}  XmcBlockStatus=1  maskContainerNames=group4  block_type=gatewayout  block_config=sysgen:gateway_out_config  block_width_w=590  block_height_w=620  block_width=620  block_height=750
  Gateway Out1 : hdlBasic/Gateway Out  inherit_from_input=off  hdl_port=off  rows=1  columns=1  UseAsDAC=off  DACChannel='1'  interface=None  automatic_assignment=on  address_offset=hex2dec('00')  intf_name=''  intf_description=''  timing_constraint=None  locs_specified=off  LOCs={}  io_standard={}  XmcBlockStatus=1  maskContainerNames=group4  block_type=gatewayout  block_config=sysgen:gateway_out_config  block_width_w=590  block_height_w=620  block_width=620  block_height=750
  Register : hdlBasic/Register  init=0  rst=off  en=off  XmcBlockStatus=1  maskContainerNames=tabcontainer1  block_type=register  block_config=sysgen:Register_config
  Register1 : hdlBasic/Register  init=0  rst=off  en=off  XmcBlockStatus=1  maskContainerNames=tabcontainer1  block_type=register  block_config=sysgen:Register_config
  Register2 : hdlBasic/Register  init=0  rst=off  en=on  XmcBlockStatus=1  maskContainerNames=tabcontainer1  block_type=register  block_config=sysgen:Register_config
  Register3 : hdlBasic/Register  init=0  rst=off  en=on  XmcBlockStatus=1  maskContainerNames=tabcontainer1  block_type=register  block_config=sysgen:Register_config
  complex_mult : hdlBasic/MCode  mfname=complex_mult  explicit_period=off  period=1  iptable={'ar','';'ai','';'br','';'bi','';'negate_bi',' 0'}  optable={'pr','off';'pi','off'}  enable_stdout=off  enable_debug=off  suppress_output=off  defparams={'negate_bi', 0}  hide_port_list={}  block_type=mcode  block_width=444  block_height=788
      settings: infoedit=Pass input values to a MATLAB function for evaluation in Xilinx fixed-point type. The input ports of the block are input arguments of the function. The output ports of the block are output arguments of the function.  block_version=8.1
  complex_mult_w_ngtd_bi : hdlBasic/MCode  mfname=complex_mult  explicit_period=off  period=1  iptable={'ar','';'ai','';'br','';'bi','';'negate_bi',' 1'}  optable={'pr','off';'pi','off'}  enable_stdout=off  enable_debug=off  suppress_output=off  defparams={'negate_bi', 1}  hide_port_list={}  block_type=mcode  block_width=444  block_height=788
      settings: infoedit=Pass input values to a MATLAB function for evaluation in Xilinx fixed-point type. The input ports of the block are input arguments of the function. The output ports of the block are output arguments of the function.  block_version=8.1
  counter : hdlBasic/MCode  mfname=fir_fsm  explicit_period=on  period=1  iptable={'reset',' false';'init',' 3'}  optable={'cnt','off';'rst','off'}  enable_stdout=off  enable_debug=off  suppress_output=off  defparams={'reset', false,'init', 3}  hide_port_list={}  block_type=mcode  block_width=444  block_height=788
      settings: infoedit=Pass input values to a MATLAB function for evaluation in Xilinx fixed-point type. The input ports of the block are input arguments of the function. The output ports of the block are output arguments of the function.  block_version=8.1
  sreg : hdlBasic/MCode  mfname=sreg  explicit_period=off  period=1  iptable={'din','';'len','4';'init','init_i'}  optable={'q','off'}  enable_stdout=off  enable_debug=off  suppress_output=off  defparams={'len',4,'init',init_i}  hide_port_list={}  block_type=mcode  block_width=444  block_height=788
      settings: infoedit=Pass input values to a MATLAB function for evaluation in Xilinx fixed-point type. The input ports of the block are input arguments of the function. The output ports of the block are output arguments of the function.  block_version=8.1
  sreg1 : hdlBasic/MCode  mfname=sreg  explicit_period=off  period=1  iptable={'din','';'len','4';'init','init_q'}  optable={'q','off'}  enable_stdout=off  enable_debug=off  suppress_output=off  defparams={'len',4,'init',init_q}  hide_port_list={}  block_type=mcode  block_width=444  block_height=788
      settings: infoedit=Pass input values to a MATLAB function for evaluation in Xilinx fixed-point type. The input ports of the block are input arguments of the function. The output ports of the block are output arguments of the function.  block_version=8.1
  I_Out : Outport  VectorParamsAs1DForOutWhenUnconnected=off
  Q_Out : Outport  Port=2  VectorParamsAs1DForOutWhenUnconnected=off
  Filter1_Coeff_I : Outport  Port=3  VectorParamsAs1DForOutWhenUnconnected=off
  Filter1_Coeff_Q : Outport  Port=4  VectorParamsAs1DForOutWhenUnconnected=off
  wires:
  Q_In/1 -> ASR1/1
  I_In/1 -> ASR/1
  ASR1/1 -> complex_mult_w_ngtd_bi/2, Delay4/1
  ASR/1 -> complex_mult_w_ngtd_bi/1, Delay/1
  Register3/1 -> Q_Out/1
  Register2/1 -> I_Out/1
  complex_mult/1 -> Register/1
  complex_mult/2 -> Register1/1
  Err_Q/1 -> complex_mult/4
  Err_I/1 -> complex_mult/3
  Gateway Out/1 -> Filter1_Coeff_I/1
  Gateway Out1/1 -> Filter1_Coeff_Q/1
  AddSub/1 -> sreg/1
  AddSub1/1 -> sreg1/1
  counter/1 -> ASR/2, ASR1/2
  counter/2 -> Delay1/1
  sreg/1 -> complex_mult_w_ngtd_bi/3, Gateway Out/1, AddSub/2
  Register/1 -> AddSub/1
  Register1/1 -> AddSub1/1
  Accumulator1/1 -> Register3/1
  complex_mult_w_ngtd_bi/2 -> Accumulator1/1
  complex_mult_w_ngtd_bi/1 -> Accumulator/1
  Delay1/1 -> Register3/2, Register2/2, Accumulator/2, Accumulator1/2
  Accumulator/1 -> Register2/1
  Delay/1 -> complex_mult/1
  Delay4/1 -> complex_mult/2
  sreg1/1 -> complex_mult_w_ngtd_bi/4, Gateway Out1/1, AddSub1/2
